simulink model "test_3way"  (R2013a)
settings: Solver=ode15s  StartTime=0.0  StopTime=8  RelTol=1e-5
libraries: fl_lib x7, nesl_utility x4, simulink x1, usask_hyd_lib x1
settings Model: Creator=tkw954  LastModifiedBy=tkw954

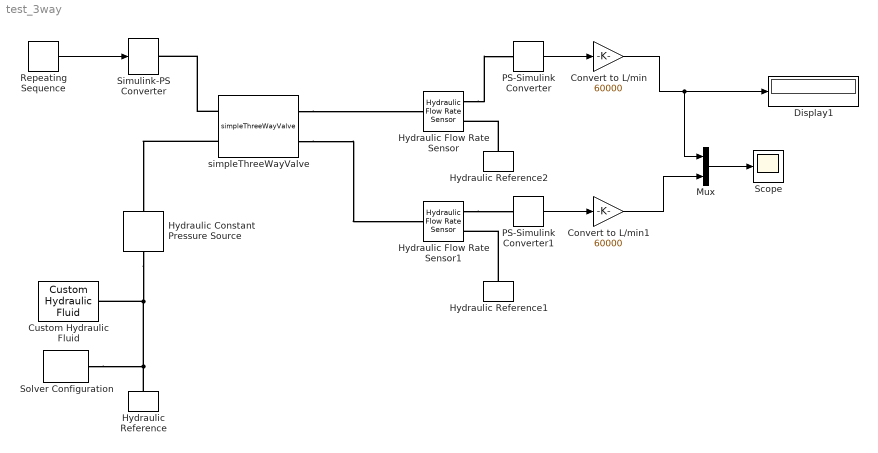
== system test_3way ==
  Convert to L/min : Gain  Gain=60000
  Convert to L/min1 : Gain  Gain=60000
  Custom Hydraulic Fluid : fl_lib/Hydraulic/Hydraulic Utilities/Custom Hydraulic Fluid  density=850 kg/m^3  viscosity_kin=18e-6 m^2/s  bulk=0.8e9 Pa  alpha=0.005  LocalVarLogging=[]
  Display1 : Display
  Hydraulic Constant Pressure Source : fl_lib/Hydraulic/Hydraulic Sources/Hydraulic Constant Pressure Source  commanded_pressure=10e6 Pa  pressure_Log=off  flow_rate_Log=off  power_Log=off  LocalVarNames=|pressure|flow_rate|power  LocalVarDescs=|Pressure differential|Flow rate|Power generated by the source  LocalVarLogging=[0 0 0]
  Hydraulic Flow Rate Sensor : fl_lib/Hydraulic/Hydraulic Sensors/Hydraulic Flow Rate Sensor  q_Log=off  p_Log=off  LocalVarNames=|q|p  LocalVarDescs=|q|p  LocalVarLogging=[0 0]
  Hydraulic Flow Rate Sensor1 : fl_lib/Hydraulic/Hydraulic Sensors/Hydraulic Flow Rate Sensor  q_Log=off  p_Log=off  LocalVarNames=|q|p  LocalVarDescs=|q|p  LocalVarLogging=[0 0]
  Hydraulic Reference : fl_lib/Hydraulic/Hydraulic Elements/Hydraulic Reference  q_Log=off  LocalVarNames=|q  LocalVarDescs=|q  LocalVarLogging=0
  Hydraulic Reference1 : fl_lib/Hydraulic/Hydraulic Elements/Hydraulic Reference  q_Log=off  LocalVarNames=|q  LocalVarDescs=|q  LocalVarLogging=0
  Hydraulic Reference2 : fl_lib/Hydraulic/Hydraulic Elements/Hydraulic Reference  q_Log=off  LocalVarNames=|q  LocalVarDescs=|q  LocalVarLogging=0
  Mux : Mux  Inputs=2
  PS-Simulink Converter : nesl_utility/PS-Simulink Converter  PhysicalDomain=network_engine_domain  SubClassName=ps_output  LeftPortType=input  RightPortType=output  PseudoPeriodic=off  Frequencies=[]  Unit=1  AffineConversion=off
  PS-Simulink Converter1 : nesl_utility/PS-Simulink Converter  PhysicalDomain=network_engine_domain  SubClassName=ps_output  LeftPortType=input  RightPortType=output  PseudoPeriodic=off  Frequencies=[]  Unit=1  AffineConversion=off
  Repeating Sequence : simulink/Sources/Repeating Sequence  rep_seq_t=[0 1 2 3 4 5 6 7 ]  rep_seq_y=[0 0 10 10 0 -10 -10 0]*1e-3
  Scope : Scope
  Simulink-PS Converter : nesl_utility/Simulink-PS Converter  PhysicalDomain=network_engine_domain  SubClassName=ps_input  LeftPortType=input  RightPortType=output  PseudoPeriodic=off  Frequencies=[]  NoiseDistribution=none  NoiseParameters=[]  Unit=1  AffineConversion=off  InputFiltering=off  SimscapeFilterOrder=1  InputFilterTimeConstant=0.001  UdotUserProvided=1
  Solver Configuration : nesl_utility/Solver Configuration  PhysicalDomain=network_engine_domain  SubClassName=solver  LeftPortType=input  RightPortType=generic  Accelerate=off  Tones=[]  Harmonics=[]  SimulateNoise=off  Profile=off  UseLocalSampling=off  EnableSwitchedLinearOptims=on  FrequencyDomain=off  UseCCode=off  UseNewInitialization=off  DoDC=off  ResidualTolerance=1e-09  UseLocalSolver=off  LocalSolverChoice=NE_BACKWARD_EULER_ADVANCER  LocalSolverSampleTime=0.001  DoFixedCost=off  MaxNonlinIter=3  MaxModeIter=2  LinearAlgebra=Sparse  DelaysMemoryBudget=1024
  simpleThreeWayValve : usask_hyd_lib/simpleThreeWayValve  A_max=50e-6  Cd=0.61  x_max=10e-3  x_OL=0  A_L=1e-9
  wires:
  PS-Simulink Converter/1 -> Convert to L/min/1
  Convert to L/min/1 -> Mux/1, Display1/1
  PS-Simulink Converter1/1 -> Convert to L/min1/1
  Convert to L/min1/1 -> Mux/2
  Mux/1 -> Scope/1
  Repeating Sequence/1 -> Simulink-PS Converter/1
  connections:
  Hydraulic Reference/LConn1 -- Solver Configuration/RConn1 -- Hydraulic Constant Pressure Source/RConn1 -- Custom Hydraulic Fluid/RConn1
  simpleThreeWayValve/RConn1 -- Hydraulic Flow Rate Sensor/LConn1
  Hydraulic Flow Rate Sensor/RConn1 -- PS-Simulink Converter/LConn1
  simpleThreeWayValve/LConn2 -- Hydraulic Constant Pressure Source/LConn1
  simpleThreeWayValve/RConn2 -- Hydraulic Flow Rate Sensor1/LConn1
  Hydraulic Flow Rate Sensor1/RConn1 -- PS-Simulink Converter1/LConn1
  simpleThreeWayValve/LConn1 -- Simulink-PS Converter/RConn1
  Hydraulic Reference1/LConn1 -- Hydraulic Flow Rate Sensor1/RConn2
  Hydraulic Reference2/LConn1 -- Hydraulic Flow Rate Sensor/RConn2
